simulink model "RL_Network"  (R2024b)
settings: Solver=VariableStepAuto  StartTime=0.0  StopTime=15e-3  RelTol=1e-3
libraries: fl_lib x5, nesl_utility x3, simulink x1
settings Model: Creator=apurvak  LastModifiedBy=apurvak

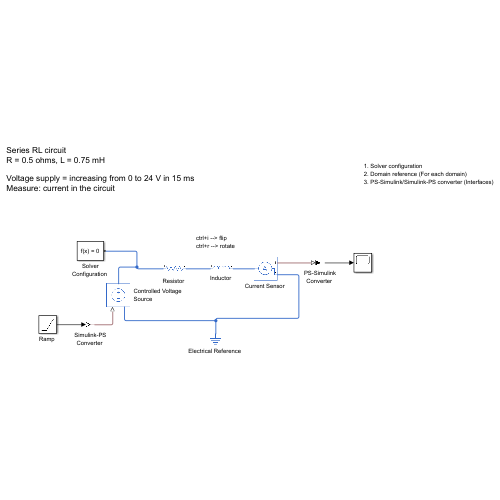
[thumbnail: Simulink's stored preview of the top-level diagram]
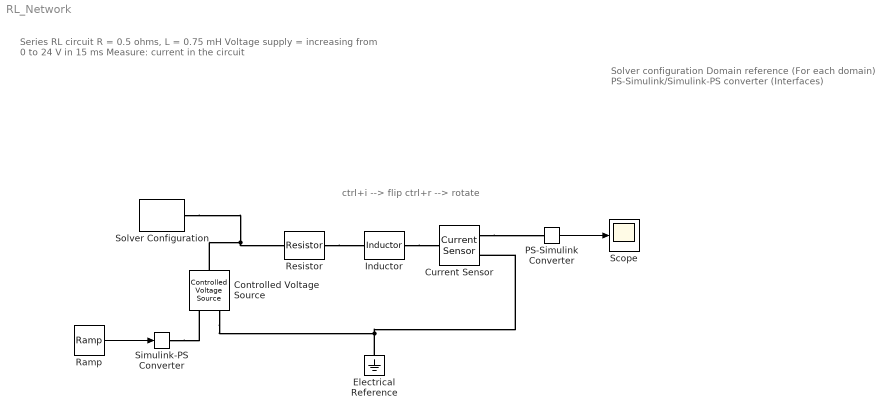
== system RL_Network ==
  note: ctrl+i --> flip
      | ctrl+r --> rotate
  note: Solver configuration
      | Domain reference (For each domain)
      | PS-Simulink/Simulink-PS converter (Interfaces)
  note: Series RL circuit
      | R = 0.5 ohms, L = 0.75 mH
      |
      | Voltage supply = increasing from 0 to 24 V in 15 ms
      | Measure: current in the circuit
  "Controlled Voltage Source " : fl_lib/Electrical/Electrical Sources/Controlled Voltage Source
  "Current Sensor " : fl_lib/Electrical/Electrical Sensors/Current Sensor
  "Electrical Reference " : fl_lib/Electrical/Electrical Elements/Electrical Reference
  "Inductor " : fl_lib/Electrical/Electrical Elements/Inductor  l=0.75 mH  r=0 Ohm  g=1e-9 1/Ohm  i_specify=off  i_priority=None  i=0 A  i_nominal_specify=off  i_nominal_value=1  i_nominal_unit=A  v_specify=off  v_priority=None  v=0 V  v_nominal_specify=off  v_nominal_value=1  v_nominal_unit=V  i_L_specify=off  i_L_priority=High  i_L=0 A  i_L_nominal_specify=off  i_L_nominal_value=1  i_L_nominal_unit=A
  "PS-Simulink Converter " : nesl_utility/PS-Simulink Converter  PhysicalDomain=network_engine_domain  SubClassName=ps_output  LeftPortType=input  RightPortType=output  PseudoPeriodic=off  Frequencies=[]  VectorFormat=inherit  Unit=inherit  AffineConversion=off
  "Ramp " : simulink/Sources/Ramp  slope=24/15e-3  start=0  InitialOutput=0
  "Resistor " : fl_lib/Electrical/Electrical Elements/Resistor  R=0.5 Ohm  i_specify=off  i_priority=None  i=0 A  i_nominal_specify=off  i_nominal_value=1  i_nominal_unit=A  v_specify=off  v_priority=None  v=0 V  v_nominal_specify=off  v_nominal_value=1  v_nominal_unit=V
  Scope : Scope
  "Simulink-PS Converter " : nesl_utility/Simulink-PS Converter  PhysicalDomain=network_engine_domain  SubClassName=ps_input  LeftPortType=input  RightPortType=output  PseudoPeriodic=off  Frequencies=[]  NoiseDistribution=none  NoiseParameters=[]  Unit=1  AffineConversion=off  FilteringAndDerivatives=provide  SimscapeFilterOrder=1  InputFilterTimeConstant=0.001  UdotUserProvided=0
  "Solver Configuration " : nesl_utility/Solver Configuration  PhysicalDomain=network_engine_domain  SubClassName=solver  LeftPortType=input  RightPortType=generic  Tones=[]  Harmonics=[]  SimulateNoise=off  Profile=off  UseLocalSampling=off  EnableSwitchedLinearOptims=on  FrequencyDomain=off  UseCCode=off  RelTol=0.001  AbsTol=0.001  MinStep=1e-09  ToWorkspace=off  RevertToSquareIcSolve=off  NumHomotopyIterations=100  PhasorMode=off  PhasorModeNumHarmonics=1  ConsistencySolver=NEWTON_XTOL_AFTER_FTOL  IndexReductionMethod=DerivativeReplacement  DoDC=off  ResidualTolerance=1e-09  ConsistencyTolSource=GLOBAL  ConsistencyAbsTol=0.001  ConsistencyRelTol=0.001  ConsistencyTolFactor=0.001  UseLocalSolver=off  LocalSolverChoice=NE_BACKWARD_EULER_ADVANCER  ResolveIndetEquations=on  FunctionEvalNumThread=1  LocalSolverSampleTime=0.001  DoFixedCost=off  MaxNonlinIter=3  MaxModeIter=2  ComputeImpulses=off  ImpulseIterations=2  LinearAlgebra=auto  LinearAlgebraNumThread=0  EquationFormulation=NE_TIME_EF  DelaysMemoryBudget=1024  AutomaticFiltering=on  FilteringTimeConstant=0.001  PartitionStorageMethod=AS_NEEDED  PartitionMemoryBudget=1024  PartitionMethod=ROBUST  MultibodyUseLocalSolver=off  MultibodyLocalSolverChoice=ODE1  MultibodyLocalSolverSampleTime=0.001
  wires:
  "PS-Simulink Converter "/1 -> Scope/1
  "Ramp "/1 -> "Simulink-PS Converter "/1
  connections:
  "Resistor "/RConn1 -- "Inductor "/LConn1
  "Solver Configuration "/RConn1 -- "Controlled Voltage Source "/LConn1 -- "Resistor "/LConn1
  "Inductor "/RConn1 -- "Current Sensor "/LConn1
  "Electrical Reference "/LConn1 -- "Controlled Voltage Source "/RConn2 -- "Current Sensor "/RConn2
  "Current Sensor "/RConn1 -- "PS-Simulink Converter "/LConn1
  "Simulink-PS Converter "/RConn1 -- "Controlled Voltage Source "/RConn1
